simulink library "PowertrainController_ul"  (R2020a)
settings: Solver=VariableStepAuto  StartTime=0.0  StopTime=10.0  RelTol=1e-3
undefined symbols (not defined in the file): best_gear, Clutch, dem_wheel_speed, dem_wheel_torque, Gear, Neg_RPM, Neg_T_eng_Nm, tau_acc, TRAN, VEH
settings Model: Creator=John Jr  LastModifiedBy=John Jr

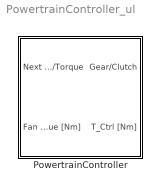
== system PowertrainController_ul ==
  PowertrainController : Subsystem

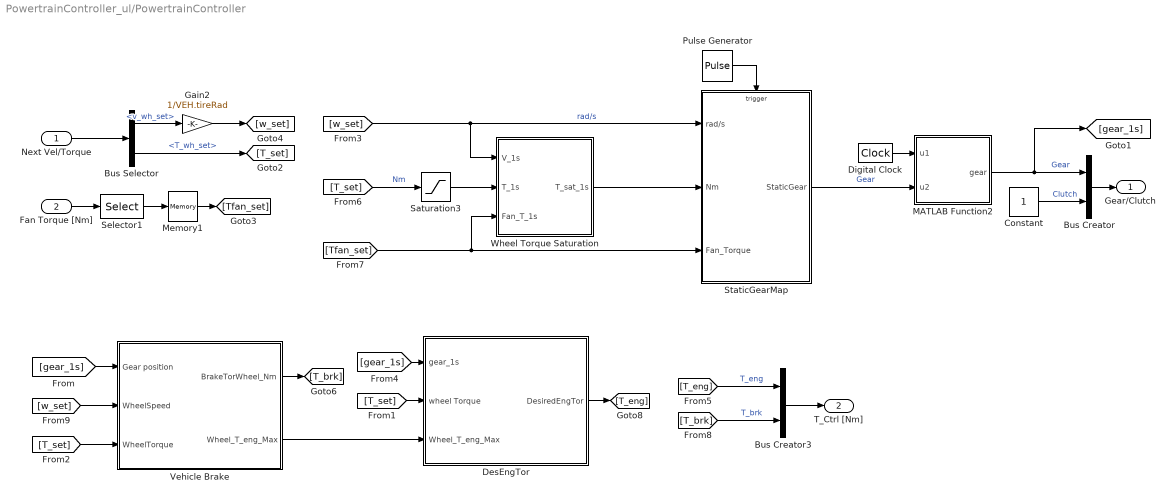
== system PowertrainController_ul/PowertrainController ==
  Next Vel/Torque : Inport
  Fan Torque [Nm] : Inport  Port=2
  Bus Creator : BusCreator  Inputs=Gear,Clutch
  Bus Creator3 : BusCreator  Inputs=2
  Bus Selector : BusSelector  OutputSignals=v_wh_set,T_wh_set
  Constant : Constant
  DesEngTor : Subsystem
  Digital Clock : DigitalClock
  Gain2 : Gain  Gain=1/VEH.tireRad
  MATLAB Function2 : MATLAB Function  TreatAsAtomicUnit=on
  Memory1 : Memory  InheritSampleTime=on
  Pulse Generator : DiscretePulseGenerator  PulseType=Time based  Period=7
  Saturation3 : Saturate  UpperLimit=inf  LowerLimit=0
  Selector1 : Selector  InputPortWidth=1  IndexOptions=Index vector (dialog)  Indices=[1]  OutputSizes=1
  StaticGearMap : Subsystem
  Vehicle Brake : Subsystem
  Wheel Torque Saturation : Subsystem
  Gear/Clutch : Outport  VectorParamsAs1DForOutWhenUnconnected=off
  T_Ctrl [Nm] : Outport  Port=2  VectorParamsAs1DForOutWhenUnconnected=off
  wires:
  MATLAB Function2/1(gear) -> [gear_1s], Bus Creator/1  "Gear"
  Pulse Generator/1 -> StaticGearMap/Trigger
  [gear_1s] -> Vehicle Brake/1(Gear position)
  [T_set] -> Saturation3/1  "Nm"
  Constant/1 -> Bus Creator/2  "Clutch"
  [w_set] -> Wheel Torque Saturation/1(V_1s), StaticGearMap/1(rad/s)  "rad/s"
  Bus Creator/1 -> Gear/Clutch/1
  [gear_1s] -> DesEngTor/1(gear_1s)
  Vehicle Brake/2(Wheel_T_eng_Max) -> DesEngTor/3(Wheel_T_eng_Max)
  Bus Creator3/1 -> T_Ctrl [Nm]/1
  Vehicle Brake/1(BrakeTorWheel_Nm) -> [T_brk]
  DesEngTor/1(DesiredEngTor) -> [T_eng]
  [T_eng] -> Bus Creator3/1  "T_eng"
  [T_brk] -> Bus Creator3/2  "T_brk"
  Next Vel/Torque/1 -> Bus Selector/1
  [T_set] -> Vehicle Brake/3(WheelTorque)
  Saturation3/1 -> Wheel Torque Saturation/2(T_1s)
  Wheel Torque Saturation/1(T_sat_1s) -> StaticGearMap/2(Nm)
  Fan Torque [Nm]/1 -> Selector1/1
  [Tfan_set] -> StaticGearMap/3(Fan_Torque), Wheel Torque Saturation/3(Fan_T_1s)
  [w_set] -> Vehicle Brake/2(WheelSpeed)
  [T_set] -> DesEngTor/2(wheel Torque)
  Selector1/1 -> Memory1/1
  Bus Selector/2 -> [T_set]  "<T_wh_set>"
  Memory1/1 -> [Tfan_set]
  Digital Clock/1 -> MATLAB Function2/1(u1)
  StaticGearMap/1(StaticGear) -> MATLAB Function2/2(u2)  "Gear"
  Bus Selector/1 -> Gain2/1  "<v_wh_set>"
  Gain2/1 -> [w_set]

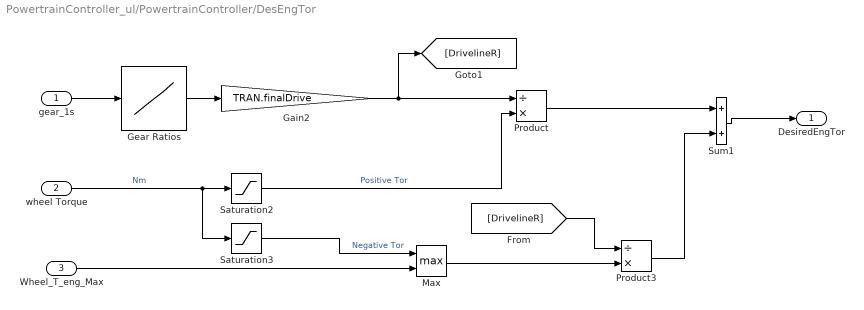
== system PowertrainController_ul/PowertrainController/DesEngTor ==
  gear_1s : Inport
  wheel Torque : Inport  Port=2
  Wheel_T_eng_Max : Inport  Port=3
  Gain2 : Gain  Gain=TRAN.finalDrive
  Gear Ratios : Lookup_n-D  NumberOfTableDimensions=1  BreakpointsForDimension1=[1:TRAN.numGears]  Table=TRAN.gears  ExtrapMethod=Clip  UseLastTableValue=on  InternalRulePriority=Speed  RndMeth=Simplest  InputSameDT=on
  Max : MinMax  Function=max  Inputs=2
  Product : Product  Inputs=/*
  Product3 : Product  Inputs=/*
  Saturation2 : Saturate  UpperLimit=inf  LowerLimit=0
  Saturation3 : Saturate  UpperLimit=0  LowerLimit=-inf
  Sum1 : Sum
  DesiredEngTor : Outport  VectorParamsAs1DForOutWhenUnconnected=off
  wires:
  Gain2/1 -> [DrivelineR], Product/1
  Product/1 -> Sum1/1
  wheel Torque/1 -> Saturation3/1, Saturation2/1  "Nm"
  Gear Ratios/1 -> Gain2/1
  gear_1s/1 -> Gear Ratios/1
  Saturation2/1 -> Product/2  "Positive Tor"
  Saturation3/1 -> Max/1  "Negative Tor"
  Sum1/1 -> DesiredEngTor/1
  Product3/1 -> Sum1/2
  Wheel_T_eng_Max/1 -> Max/2
  Max/1 -> Product3/2
  [DrivelineR] -> Product3/1

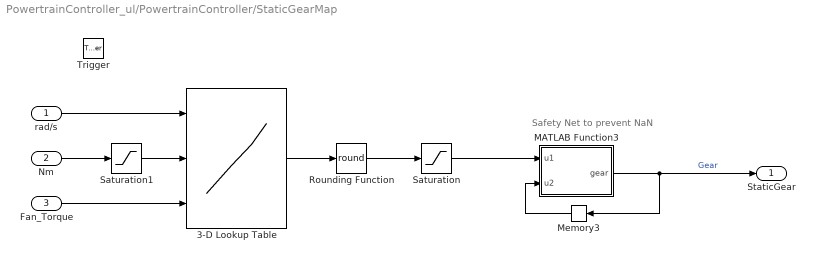
== system PowertrainController_ul/PowertrainController/StaticGearMap ==
  note: Safety Net to prevent NaN
  rad/s : Inport
  Nm : Inport  Port=2
  Fan_Torque : Inport  Port=3
  Trigger : TriggerPort  VariantControl=Variant  PortDimensions=1
  3-D Lookup Table : Lookup_n-D  NumberOfTableDimensions=3  BreakpointsForDimension1=dem_wheel_speed  BreakpointsForDimension2=dem_wheel_torque  BreakpointsForDimension3=tau_acc  Table=best_gear  InternalRulePriority=Speed  RndMeth=Simplest  InputSameDT=on
  MATLAB Function3 : MATLAB Function  TreatAsAtomicUnit=on
  Memory3 : Memory  InitialCondition=11  InheritSampleTime=on
  Rounding Function : Rounding  Operator=round
  Saturation : Saturate  UpperLimit=12  LowerLimit=1
  Saturation1 : Saturate  UpperLimit=inf  LowerLimit=0
  StaticGear : Outport  VectorParamsAs1DForOutWhenUnconnected=off
  wires:
  Fan_Torque/1 -> 3-D Lookup Table/3
  Rounding Function/1 -> Saturation/1
  Saturation1/1 -> 3-D Lookup Table/2
  Nm/1 -> Saturation1/1
  rad/s/1 -> 3-D Lookup Table/1
  3-D Lookup Table/1 -> Rounding Function/1
  Memory3/1 -> MATLAB Function3/2(u2)
  Saturation/1 -> MATLAB Function3/1(u1)
  MATLAB Function3/1(gear) -> StaticGear/1, Memory3/1  "Gear"

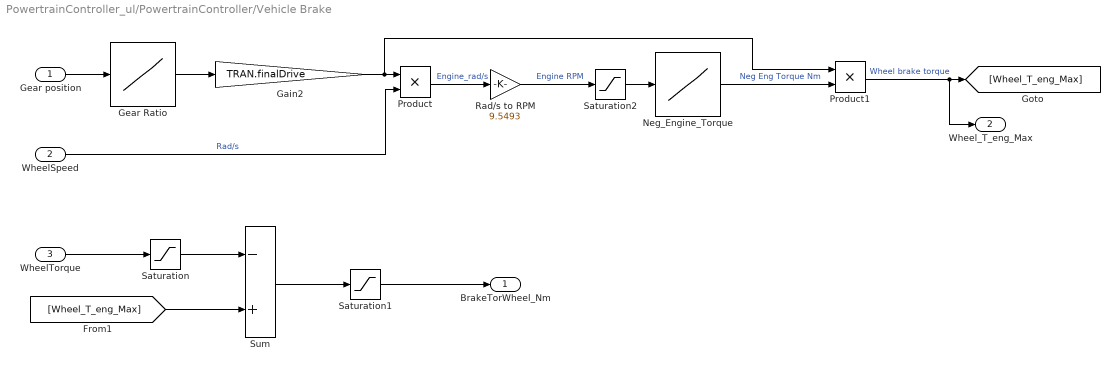
== system PowertrainController_ul/PowertrainController/Vehicle Brake ==
  Gear position : Inport
  WheelSpeed : Inport  Port=2
  WheelTorque : Inport  Port=3
  Gain2 : Gain  Gain=TRAN.finalDrive
  Gear Ratio : Lookup_n-D  NumberOfTableDimensions=1  BreakpointsForDimension1=[1 2 3 4 5 6 7 8 9 10 11 12]  BreakpointsForDimension2=[1:3]  Table=[11.73 9.21 7.09 5.57 4.34 3.41 2.69 2.12 1.63 1.28 1 0.7850]  InternalRulePriority=Speed  RndMeth=Simplest  InputSameDT=on
  Neg_Engine_Torque : Lookup_n-D  NumberOfTableDimensions=1  BreakpointsForDimension1=Neg_RPM  BreakpointsForDimension2=[1:3]  Table=Neg_T_eng_Nm  InternalRulePriority=Speed  RndMeth=Simplest  InputSameDT=on
  Product : Product
  Product1 : Product
  Rad/s to RPM : Gain  Gain=9.5493
  Saturation : Saturate  UpperLimit=0  LowerLimit=-inf
  Saturation1 : Saturate  UpperLimit=inf  LowerLimit=0
  Saturation2 : Saturate  UpperLimit=2100  LowerLimit=0
  Sum : Sum  Inputs=-+
  BrakeTorWheel_Nm : Outport  VectorParamsAs1DForOutWhenUnconnected=off
  Wheel_T_eng_Max : Outport  Port=2  VectorParamsAs1DForOutWhenUnconnected=off
  wires:
  Rad/s to RPM/1 -> Saturation2/1  "Engine RPM"
  Neg_Engine_Torque/1 -> Product1/2  "Neg Eng Torque Nm"
  Gear position/1 -> Gear Ratio/1
  Gear Ratio/1 -> Gain2/1
  Gain2/1 -> Product1/1, Product/1
  WheelSpeed/1 -> Product/2  "Rad/s"
  Product/1 -> Rad/s to RPM/1  "Engine_rad/s"
  Product1/1 -> Wheel_T_eng_Max/1, [Wheel_T_eng_Max]  "Wheel brake torque"
  WheelTorque/1 -> Saturation/1
  [Wheel_T_eng_Max] -> Sum/2
  Saturation/1 -> Sum/1
  Sum/1 -> Saturation1/1
  Saturation1/1 -> BrakeTorWheel_Nm/1
  Saturation2/1 -> Neg_Engine_Torque/1

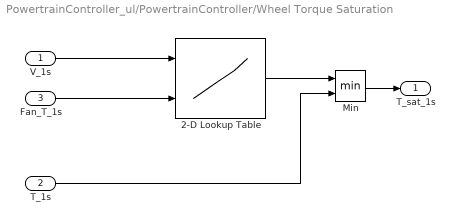
== system PowertrainController_ul/PowertrainController/Wheel Torque Saturation ==
  V_1s : Inport
  T_1s : Inport  Port=2
  Fan_T_1s : Inport  Port=3
  2-D Lookup Table : Lookup_n-D  BreakpointsForDimension1=dem_wheel_speed  BreakpointsForDimension2=tau_acc  Table=WheelTorque_Max'  InternalRulePriority=Speed  RndMeth=Simplest  InputSameDT=on
  Min : MinMax  Inputs=2
  T_sat_1s : Outport  VectorParamsAs1DForOutWhenUnconnected=off
  wires:
  V_1s/1 -> 2-D Lookup Table/1
  Fan_T_1s/1 -> 2-D Lookup Table/2
  2-D Lookup Table/1 -> Min/1
  T_1s/1 -> Min/2
  Min/1 -> T_sat_1s/1

== matlab function PowertrainController_ul/PowertrainController/StaticGearMap/MATLAB Function3 ==
  data: u1 input; gear output; u2 input
function gear = fcn(u1, u2)
if isnan(u1)
    gear=u2;
else
    gear=u1;
end

== matlab function PowertrainController_ul/PowertrainController/MATLAB Function2 ==
  data: u1 input; gear output; u2 input
function gear = fcn(u1, u2)
if u1 <= 7 
    gear=11;
else
    gear=u2;
end
